simulink model "stumbler_simulation"  (Simulink 9.3)
settings: Solver=ode45  StartTime=0.0  StopTime=1  RelTol=1e-3  EnableMultiTasking=on
StopFcn:
  | plot_stumbler
settings Model: Creator=Marleen  LastModifiedBy=SID-Drebbelweg
settings DataIOCC: LimitDataPoints=on
settings OptimizationCC: InitFltsAndDblsToZero=on
settings DebuggingCC: SaveWithParameterizedLinksMsg=none  SignalResolutionControl=TryResolveAllWithWarning  SolverPrmCheckMsg=warning  MultiTaskDSMMsg=warning  MultiTaskCondExecSysMsg=none
settings GRTTargetCC: TargetFcnLib=ansi_tfl_tmw.mat

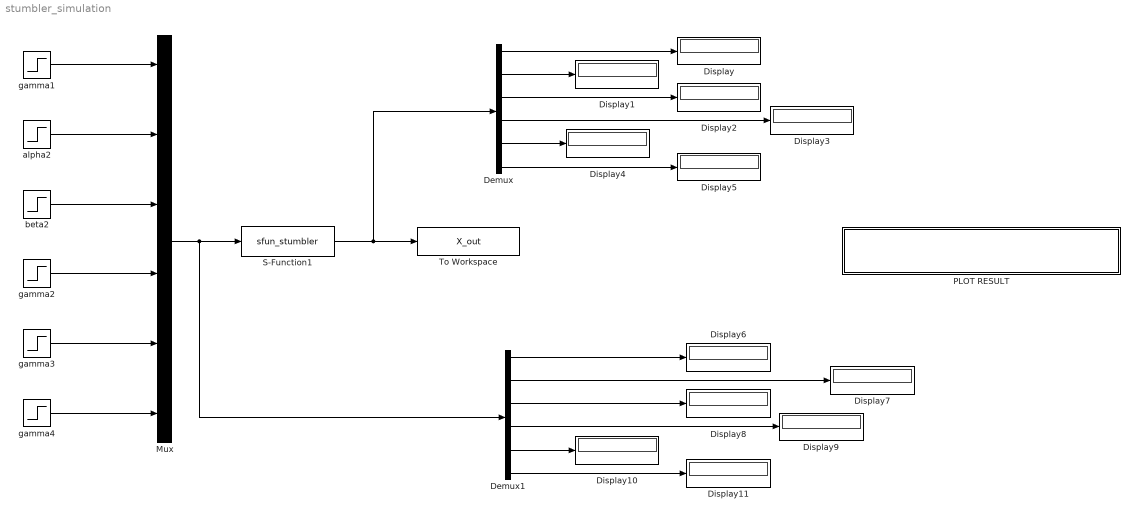
== system stumbler_simulation ==
  Demux : Demux  Outputs=6
  Demux1 : Demux  Outputs=6
  Display{,1..11} (12 alike) : Display
  Mux : Mux  Inputs=6
  PLOT RESULT : Subsystem
      settings: OpenFcn=plot_stumbler
      mask Display: disp('DoubleClick to Animate')
  S-Function1 : S-Function  FunctionName=sfun_stumbler  SFunctionDeploymentMode=off  EnableBusSupport=off
  To Workspace : ToWorkspace  VariableName=X_out  SaveFormat=Structure With Time  SampleTime=0.01
  alpha2 : Step  Time=0  After=0  SampleTime=0
  beta2 : Step  Time=0  After=0  SampleTime=0
  gamma1 : Step  Time=0  After=0  SampleTime=0
  gamma2 : Step  Time=0.7  Before=10  After=0  SampleTime=0
  gamma3 : Step  Time=0.6  After=10  SampleTime=0
  gamma4 : Step  Time=0  After=0  SampleTime=0
  wires:
  S-Function1/1 -> To Workspace/1, Demux/1
  Mux/1 -> Demux1/1, S-Function1/1
  gamma1/1 -> Mux/1
  alpha2/1 -> Mux/2
  beta2/1 -> Mux/3
  gamma2/1 -> Mux/4
  gamma3/1 -> Mux/5
  gamma4/1 -> Mux/6
  Demux/1 -> Display/1
  Demux/2 -> Display1/1
  Demux/3 -> Display2/1
  Demux/4 -> Display3/1
  Demux/5 -> Display4/1
  Demux/6 -> Display5/1
  Demux1/4 -> Display9/1
  Demux1/3 -> Display8/1
  Demux1/2 -> Display7/1
  Demux1/6 -> Display11/1
  Demux1/5 -> Display10/1
  Demux1/1 -> Display6/1

== system stumbler_simulation/PLOT RESULT ==
